simulink model "MI6FS_HE_6PhS"  (R2023a)
settings: Solver=FixedStepAuto  StartTime=0  StopTime=L  FixedStep=Ts  RelTol=1e-3
values from neighbouring files (symbols this model uses):
  A = exp(j*pi/3)    [Parameters.m]
  deg = 0    [Parameters.m]
  FV = 9.8    [Parameters.m]
  J = 0.0243    [Parameters.m]
  Lrr = [((1/3*Lm)+Llr) 1/6*Lm -1/6*Lm -1/3*Lm -1/6*Lm 1/6*Lm;        1/6*Lm ((1/3*Lm)+Llr) 1/6*Lm -1/6*Lm -1/3*Lm -1/6*Lm;        -1/6*Lm 1/6*Lm ((1/3*Lm)+Llr) 1/6*Lm -1/6*Lm -1/3*Lm;        -1/3*Lm -1/6*Lm 1/6*Lm ((1/3*Lm)+Llr) 1/6*Lm -1/6*Lm;        -1/6*Lm -1/3*Lm -1/6*Lm 1/6*Lm ((1/3*Lm)+Llr) 1/6*Lm;        1/6*Lm -1/6*Lm -1/3*Lm -1/6*Lm 1/6*Lm ((1/3*Lm)+Llr)]    [Parameters.m]
  Lrs = transpose(Lsr)    [Parameters.m]
  Lsr = [0 (pi/3) 2*(pi/3) 3*(pi/3) 4*(pi/3) 5*(pi/3);        -(pi/3) 0 (pi/3) 2*(pi/3) 3*(pi/3) 4*(pi/3);        -2*(pi/3) -(pi/3) 0 (pi/3) 2*(pi/3) 3*(pi/3);        -3*(pi/3) -2*(pi/3) -(pi/3) 0 (pi/3) 2*(pi/3);        -4*(pi/3) -3*(pi/3) -2*(pi/3) -(pi/3) 0 (pi/3);        -5*(pi/3) -4*(pi/3) -3*(pi/3) -2*(pi/3) -(pi/3) 0]    [Parameters.m]
  Lss = [((1/3*Lm)+Lls) 1/6*Lm -1/6*Lm -1/3*Lm -1/6*Lm 1/6*Lm;        1/6*Lm ((1/3*Lm)+Lls) 1/6*Lm -1/6*Lm -1/3*Lm -1/6*Lm;        -1/6*Lm 1/6*Lm ((1/3*Lm)+Lls) 1/6*Lm -1/6*Lm -1/3*Lm;        -1/3*Lm -1/6*Lm 1/6*Lm ((1/3*Lm)+Lls) 1/6*Lm -1/6*Lm;        -1/6*Lm -1/3*Lm -1/6*Lm 1/6*Lm ((1/3*Lm)+Lls) 1/6*Lm;        1/6*Lm -1/6*Lm -1/3*Lm -1/6*Lm 1/6*Lm ((1/3*Lm)+Lls)]    [Parameters.m]
  Lto = 0    [Parameters.m]
  Msr = (1/3)*Lm    (= 0.0620333333333)    [Parameters.m]
  p = 2    [Parameters.m]
  Rcore = 811    [Parameters.m]
  Rrr = Rr*eye(6,6)    [Parameters.m]
  Rss = Rs*eye(6,6)    [Parameters.m]
  Tav = 0.23    [Parameters.m]
  Ts = 1/Fs    (= 1e-05)    [Parameters.m]
  Us = sqrt(2)*180    [Parameters.m]
undefined symbols (not defined in the file or in its folder): DiscIntNeverNeededParam, j
libraries: spsFourierLib x84, spsVoltageMeasurementLib x13, spsACVoltageSourceLib x6, spsControlledCurrentSourceLib x6, spsCurrentMeasurementLib x6, spsSeriesRLCBranchLib x6, spsSequenceAnalyzerLib x6, sharedutil x5, eeRmsMeasurement x2, eeGeneralControl x1, spsSequenceAnalyzerPhasorLib x1, spsabctoAlphaBetaZeroLib x1
(part 2 of 3)

== system MI6FS_HE_6PhS/Phase System/Subsystem12 ==
  abc : Inport
  -wt : Subsystem
  Demux : Demux  Outputs=3
  Demux1 : Demux  Outputs=3
  Demux2 : Demux  Outputs=3
  Display : Display
  Display1 : Display
  Display2 : Display
  Divide : Product  Inputs=*/
  Exp : Math
  Gain : Gain  Gain=j
  Gain1 : Gain  Gain=pi/180
  Magnitude-Angle to Complex1 : MagnitudeAngleToComplex
  Minus : Sum  Inputs=+-
  Product : Product
  Scope : Scope
  Sequence Analyzer1 : spsSequenceAnalyzerLib/Sequence Analyzer  Freq=50  n=1  seq=Positive Negative Zero  InInit=[0, 0]  Ts=Ts
  P : Outport
  N : Outport  Port=2
  0 : Outport  Port=3
  |u| : Outport  Port=4
  <u : Outport  Port=5
  wires:
  Product/1 -> Scope/1
  Gain/1 -> Exp/1
  -wt/1(-wt) -> Gain/1
  Exp/1 -> Product/1
  Demux1/1 -> Minus/2
  Demux1/2 -> Minus/1
  Demux2/2 -> Divide/1
  Demux2/1 -> Divide/2
  Minus/1 -> Display2/1
  Divide/1 -> Display1/1
  Demux/3 -> 0/1
  Demux/2 -> N/1, Product/2
  Gain1/1 -> Demux1/1, Magnitude-Angle to Complex1/2
  Demux/1 -> P/1
  abc/1 -> Sequence Analyzer1/1
  Sequence Analyzer1/1 -> |u|/1, Magnitude-Angle to Complex1/1, Demux2/1
  Sequence Analyzer1/2 -> <u/1, Gain1/1
  Magnitude-Angle to Complex1/1 -> Display/1, Demux/1

== system MI6FS_HE_6PhS/Phase System/Subsystem13 ==
  abc : Inport
  -wt : Subsystem
  Demux : Demux  Outputs=3
  Demux1 : Demux  Outputs=3
  Demux2 : Demux  Outputs=3
  Display : Display
  Display1 : Display
  Display2 : Display
  Divide : Product  Inputs=*/
  Exp : Math
  Gain : Gain  Gain=j
  Gain1 : Gain  Gain=pi/180
  Magnitude-Angle to Complex1 : MagnitudeAngleToComplex
  Minus : Sum  Inputs=+-
  Product : Product
  Scope : Scope
  Sequence Analyzer1 : spsSequenceAnalyzerLib/Sequence Analyzer  Freq=50  n=1  seq=Positive Negative Zero  InInit=[0, 0]  Ts=Ts
  P : Outport
  N : Outport  Port=2
  0 : Outport  Port=3
  |u| : Outport  Port=4
  <u : Outport  Port=5
  wires:
  Magnitude-Angle to Complex1/1 -> Demux/1, Display/1
  Sequence Analyzer1/2 -> Gain1/1, <u/1
  Sequence Analyzer1/1 -> Demux2/1, Magnitude-Angle to Complex1/1, |u|/1
  abc/1 -> Sequence Analyzer1/1
  Demux/1 -> P/1
  Gain1/1 -> Magnitude-Angle to Complex1/2, Demux1/1
  Demux/2 -> Product/2, N/1
  Demux/3 -> 0/1
  Divide/1 -> Display1/1
  Minus/1 -> Display2/1
  Demux2/1 -> Divide/2
  Demux2/2 -> Divide/1
  Demux1/2 -> Minus/1
  Demux1/1 -> Minus/2
  Exp/1 -> Product/1
  -wt/1(-wt) -> Gain/1
  Gain/1 -> Exp/1
  Product/1 -> Scope/1

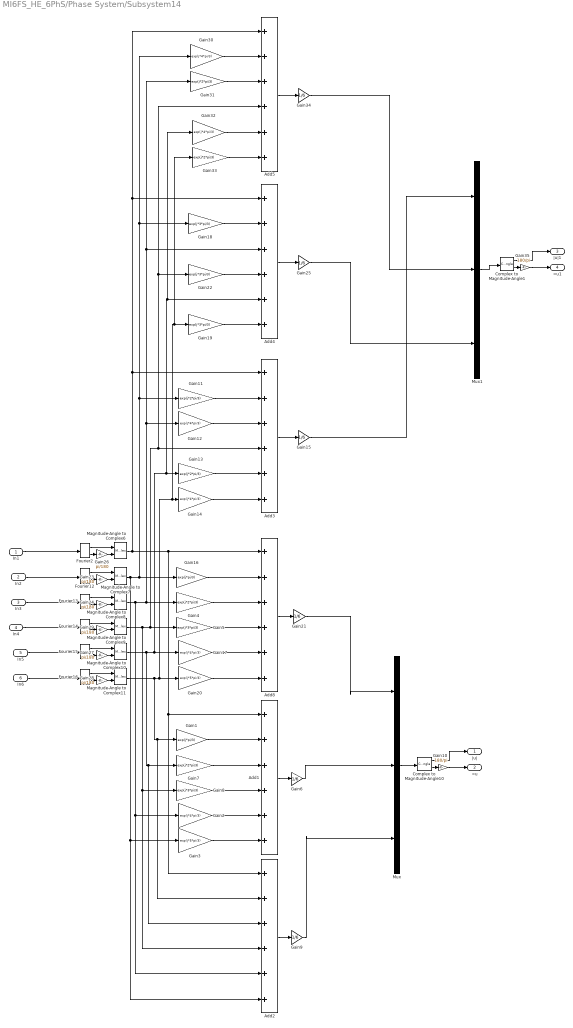
== system MI6FS_HE_6PhS/Phase System/Subsystem14 ==
  In1 : Inport
  In2 : Inport  Port=2
  In3 : Inport  Port=3
  In4 : Inport  Port=4
  In5 : Inport  Port=5
  In6 : Inport  Port=6
  Add{1..5,8} (6 alike) : Sum  Inputs=++++++
  Complex to Magnitude-Angle1 : ComplexToMagnitudeAngle
  Complex to Magnitude-Angle10 : ComplexToMagnitudeAngle
  Fourier{2,12..16} (6 alike) : spsFourierLib/Fourier  Freq=50  n=1  InInit=[0, 0]  Ts=Ts
  Gain1 : Gain  Gain=exp(j*pi/3)
  Gain10 : Gain  Gain=180/pi
  Gain{4,7,11,13,31,33} (6 alike) : Gain  Gain=exp(j*2*pi/3)
  Gain{2,12,14,17,30,32} (6 alike) : Gain  Gain=exp(j*4*pi/3)
  Gain{6,9,15,21,25,34} (6 alike) : Gain  Gain=1/6
  Gain16 : Gain  Gain=exp(j*pi/3)
  Gain{5,8,18..19,22} (5 alike) : Gain  Gain=exp(j*3*pi/3)
  Gain20 : Gain  Gain=exp(j*5*pi/3)
  Gain{23..24,26..29} (6 alike) : Gain  Gain=pi/180
  Gain3 : Gain  Gain=exp(j*5*pi/3)
  Gain35 : Gain  Gain=180/pi
  Magnitude-Angle to Complex{6..11} (6 alike) : MagnitudeAngleToComplex
  Mux : Mux  Inputs=3
  Mux1 : Mux  Inputs=3
  |u| : Outport
  <u : Outport  Port=2
  |u|1 : Outport  Port=3
  <u1 : Outport  Port=4
  wires:
  Gain16/1 -> Add8/2
  Fourier14/2 -> Gain29/1
  Fourier12/2 -> Gain23/1
  Gain27/1 -> Magnitude-Angle to Complex10/2
  Fourier2/2 -> Gain26/1
  Fourier14/1 -> Magnitude-Angle to Complex9/1
  In6/1 -> Fourier16/1
  Magnitude-Angle to Complex7/1 -> Add2/6, Gain3/1, Gain30/1, Gain18/1, Gain11/1, Gain16/1
  Gain28/1 -> Magnitude-Angle to Complex11/2
  In4/1 -> Fourier14/1
  Fourier16/1 -> Magnitude-Angle to Complex11/1
  Fourier2/1 -> Magnitude-Angle to Complex6/1
  Gain4/1 -> Add8/3
  Gain5/1 -> Add8/4
  Magnitude-Angle to Complex10/1 -> Add2/3, Gain7/1, Gain13/1, Gain32/1, Add4/5, Gain17/1
  Magnitude-Angle to Complex9/1 -> Add2/4, Gain8/1, Add5/4, Gain22/1, Add3/4, Gain5/1
  Fourier13/2 -> Gain24/1
  Gain29/1 -> Magnitude-Angle to Complex9/2
  Gain17/1 -> Add8/5
  Gain20/1 -> Add8/6
  In1/1 -> Fourier2/1
  In3/1 -> Fourier13/1
  Fourier16/2 -> Gain28/1
  Fourier15/2 -> Gain27/1
  Fourier15/1 -> Magnitude-Angle to Complex10/1
  Gain23/1 -> Magnitude-Angle to Complex7/2
  Gain24/1 -> Magnitude-Angle to Complex8/2
  Gain26/1 -> Magnitude-Angle to Complex6/2
  Fourier13/1 -> Magnitude-Angle to Complex8/1
  Fourier12/1 -> Magnitude-Angle to Complex7/1
  Add8/1 -> Gain21/1
  Magnitude-Angle to Complex8/1 -> Add2/5, Gain2/1, Gain31/1, Add4/3, Gain12/1, Gain4/1
  In5/1 -> Fourier15/1
  In2/1 -> Fourier12/1
  Gain21/1 -> Mux/1
  Gain3/1 -> Add1/6
  Gain8/1 -> Add1/4
  Gain7/1 -> Add1/3
  Gain2/1 -> Add1/5
  Add1/1 -> Gain6/1
  Gain1/1 -> Add1/2
  Magnitude-Angle to Complex6/1 -> Add5/1, Add4/1, Add3/1, Add2/1, Add1/1, Add8/1
  Gain6/1 -> Mux/2
  Gain9/1 -> Mux/3
  Add2/1 -> Gain9/1
  Complex to Magnitude-Angle10/2 -> Gain10/1
  Mux/1 -> Complex to Magnitude-Angle10/1
  Gain10/1 -> <u/1
  Complex to Magnitude-Angle10/1 -> |u|/1
  Gain11/1 -> Add3/2
  Gain12/1 -> Add3/3
  Gain13/1 -> Add3/5
  Gain14/1 -> Add3/6
  Add3/1 -> Gain15/1
  Gain18/1 -> Add4/2
  Gain22/1 -> Add4/4
  Gain19/1 -> Add4/6
  Add4/1 -> Gain25/1
  Gain30/1 -> Add5/2
  Gain31/1 -> Add5/3
  Gain32/1 -> Add5/5
  Gain33/1 -> Add5/6
  Magnitude-Angle to Complex11/1 -> Add2/2, Gain1/1, Gain19/1, Gain33/1, Gain14/1, Gain20/1
  Add5/1 -> Gain34/1
  Complex to Magnitude-Angle1/1 -> |u|1/1
  Gain35/1 -> <u1/1
  Complex to Magnitude-Angle1/2 -> Gain35/1
  Mux1/1 -> Complex to Magnitude-Angle1/1
  Gain15/1 -> Mux1/1
  Gain34/1 -> Mux1/2
  Gain25/1 -> Mux1/3

== system MI6FS_HE_6PhS/Phase System/Subsystem15 ==
  In1 : Inport
  In2 : Inport  Port=2
  In3 : Inport  Port=3
  Add{1..6} (6 alike) : Sum  Inputs=3
  Add7 : Sum  Inputs=2
  Complex to Magnitude-Angle : ComplexToMagnitudeAngle
  Complex to Magnitude-Angle1 : ComplexToMagnitudeAngle
  Complex to Magnitude-Angle2 : ComplexToMagnitudeAngle
  Display{,1..5} (6 alike) : Display
  Gain{1,5,8,16} (4 alike) : Gain  Gain=exp(j*4*pi/3)
  Gain10 : Gain  Gain=180/pi
  Gain11 : Gain  Gain=180/pi
  Gain12 : Gain  Gain=180/pi
  Gain13 : Gain  Gain=2/3
  Gain{2,4,6,17} (4 alike) : Gain  Gain=exp(j*2*pi/3)
  Gain19 : Gain  Gain=-1/2
  Gain22 : Gain  Gain=2/3
  Gain3 : Gain  Gain=-sqrt(3)/2
  Gain7 : Gain  Gain=-1/2
  Gain9 : Gain  Gain=sqrt(3)/2
  Out1 : Outport
  Out2 : Outport  Port=2
  wires:
  Add1/1 -> Complex to Magnitude-Angle/1, Add6/1
  Gain16/1 -> Add5/2
  In1/1 -> Gain17/1, Gain8/1, Gain2/1, Gain5/1, Add1/1
  Add5/1 -> Complex to Magnitude-Angle2/1, Gain19/1
  In2/1 -> Gain16/1, Gain6/1, Gain1/1, Gain4/1, Add1/2
  Gain17/1 -> Add5/1
  In3/1 -> Add5/3, Add2/3, Add3/3, Add4/3, Add1/3
  Gain4/1 -> Add4/2
  Add4/1 -> Complex to Magnitude-Angle1/1, Gain7/1
  Gain19/1 -> Add6/3
  Gain7/1 -> Add6/2
  Gain5/1 -> Add4/1
  Gain6/1 -> Add2/2
  Gain8/1 -> Add2/1
  Gain1/1 -> Add3/2
  Add3/1 -> Gain3/1
  Gain2/1 -> Add3/1
  Add2/1 -> Gain9/1
  Gain9/1 -> Add7/1
  Gain3/1 -> Add7/2
  Complex to Magnitude-Angle/1 -> Display/1
  Gain10/1 -> Display1/1
  Complex to Magnitude-Angle/2 -> Gain10/1
  Gain11/1 -> Display3/1
  Complex to Magnitude-Angle1/2 -> Gain11/1
  Complex to Magnitude-Angle1/1 -> Display2/1
  Gain12/1 -> Display5/1
  Complex to Magnitude-Angle2/2 -> Gain12/1
  Complex to Magnitude-Angle2/1 -> Display4/1
  Add6/1 -> Gain22/1
  Gain22/1 -> Out1/1
  Gain13/1 -> Out2/1
  Add7/1 -> Gain13/1

== system MI6FS_HE_6PhS/Phase System/Subsystem16 ==
  In1 : Inport
  In2 : Inport  Port=2
  In3 : Inport  Port=3
  In4 : Inport  Port=4
  In5 : Inport  Port=5
  In6 : Inport  Port=6
  Add1 : Sum  Inputs=6
  Display{,2..3,100..111} (15 alike) : Display
  Divide : Product  Inputs=*/
  Fourier{32..37} (6 alike) : spsFourierLib/Fourier  Freq=50  n=1  InInit=[0, 0]  Ts=Ts
  Gain15 : Gain  Gain=1/6
  Max of Elements : MinMax  Function=max
  Minus{,1..5} (6 alike) : Sum  Inputs=+-
  Mux : Mux  Inputs=6
  Out1 : Outport
  Out2 : Outport  Port=2
  wires:
  Fourier32/1 -> Minus1/1, Add1/2, Display102/1
  Fourier32/2 -> Display103/1
  Add1/1 -> Gain15/1
  Fourier33/2 -> Display105/1
  Fourier33/1 -> Minus2/1, Add1/3, Display104/1
  Fourier34/1 -> Display106/1, Minus3/1, Add1/4
  Fourier36/1 -> Display110/1, Minus5/1, Add1/6
  Fourier37/1 -> Display100/1, Minus/1, Add1/1
  Fourier35/1 -> Display108/1, Minus4/1, Add1/5
  In4/1 -> Fourier34/1
  Fourier35/2 -> Display109/1
  Fourier37/2 -> Display101/1
  Fourier36/2 -> Display111/1
  Fourier34/2 -> Display107/1
  Gain15/1 -> Divide/2, Out1/1, [avg]
  In6/1 -> Fourier36/1
  In3/1 -> Fourier33/1
  In5/1 -> Fourier35/1
  In1/1 -> Fourier37/1
  In2/1 -> Fourier32/1
  [avg] -> Minus1/2, Minus/2, Minus2/2, Minus5/2, Minus4/2, Minus3/2
  Mux/1 -> Max of Elements/1, Display2/1
  Minus5/1 -> Mux/6
  Minus4/1 -> Mux/5
  Minus3/1 -> Mux/4
  Minus2/1 -> Mux/3
  Minus1/1 -> Mux/2
  Minus/1 -> Mux/1
  Max of Elements/1 -> Display3/1, Divide/1
  Divide/1 -> Out2/1, Display/1

== system MI6FS_HE_6PhS/Phase System/Subsystem17 ==
  In6 : Inport
  In1 : Inport  Port=2
  In2 : Inport  Port=3
  In3 : Inport  Port=4
  In4 : Inport  Port=5
  In5 : Inport  Port=6
  Add : Sum  Inputs=6
  Add1 : Sum  Inputs=6
  Gain : Gain  Gain=1/3
  Gain1 : Gain  Gain=cos(3*pi/3)
  Gain2 : Gain  Gain=cos(4*pi/3)
  Gain23 : Gain  Gain=cos(pi/3)
  Gain24 : Gain  Gain=cos(2*pi/3)
  Gain3 : Gain  Gain=cos(5*pi/3)
  Gain4 : Gain  Gain=1/3
  Gain5 : Gain  Gain=sin(3*pi/3)
  Gain6 : Gain  Gain=sin(4*pi/3)
  Gain7 : Gain  Gain=sin(pi/3)
  Gain8 : Gain  Gain=sin(2*pi/3)
  Gain9 : Gain  Gain=sin(5*pi/3)
  Out1 : Outport
  Out2 : Outport  Port=2
  wires:
  Gain23/1 -> Add/2
  Gain24/1 -> Add/3
  Add/1 -> Gain/1
  Gain1/1 -> Add/4
  Gain2/1 -> Add/5
  Gain3/1 -> Add/6
  In6/1 -> Add/1
  Gain/1 -> Out1/1
  Gain5/1 -> Add1/4
  In2/1 -> Gain8/1, Gain24/1
  In3/1 -> Gain5/1, Gain1/1
  In5/1 -> Gain9/1, Gain3/1
  In4/1 -> Gain6/1, Gain2/1
  Gain7/1 -> Add1/2
  In1/1 -> Gain7/1, Gain23/1
  Add1/1 -> Gain4/1
  Gain4/1 -> Out2/1
  Gain9/1 -> Add1/6
  Gain8/1 -> Add1/3
  Gain6/1 -> Add1/5

== system MI6FS_HE_6PhS/Phase System/Subsystem18 ==
  In6 : Inport
  In1 : Inport  Port=2
  In2 : Inport  Port=3
  In3 : Inport  Port=4
  In4 : Inport  Port=5
  In5 : Inport  Port=6
  Add : Sum  Inputs=6
  Add1 : Sum  Inputs=6
  Gain : Gain  Gain=1/3
  Gain1 : Gain  Gain=cos(3*pi/3)
  Gain2 : Gain  Gain=cos(4*pi/3)
  Gain23 : Gain  Gain=cos(pi/3)
  Gain24 : Gain  Gain=cos(2*pi/3)
  Gain3 : Gain  Gain=cos(5*pi/3)
  Gain4 : Gain  Gain=1/3
  Gain5 : Gain  Gain=sin(3*pi/3)
  Gain6 : Gain  Gain=sin(4*pi/3)
  Gain7 : Gain  Gain=sin(pi/3)
  Gain8 : Gain  Gain=sin(2*pi/3)
  Gain9 : Gain  Gain=sin(5*pi/3)
  Out1 : Outport
  Out2 : Outport  Port=2
  wires:
  Gain6/1 -> Add1/5
  Gain8/1 -> Add1/3
  Gain9/1 -> Add1/6
  Gain4/1 -> Out2/1
  Add1/1 -> Gain4/1
  In1/1 -> Gain23/1, Gain7/1
  Gain7/1 -> Add1/2
  In4/1 -> Gain2/1, Gain6/1
  In5/1 -> Gain3/1, Gain9/1
  In3/1 -> Gain1/1, Gain5/1
  In2/1 -> Gain24/1, Gain8/1
  Gain5/1 -> Add1/4
  Gain/1 -> Out1/1
  In6/1 -> Add/1
  Gain3/1 -> Add/6
  Gain2/1 -> Add/5
  Gain1/1 -> Add/4
  Add/1 -> Gain/1
  Gain24/1 -> Add/3
  Gain23/1 -> Add/2

== system MI6FS_HE_6PhS/Phase System/Subsystem19 ==
  In1 : Inport
  In2 : Inport  Port=2
  In3 : Inport  Port=3
  In4 : Inport  Port=4
  In5 : Inport  Port=5
  In6 : Inport  Port=6
  Complex to Magnitude-Angle{2..7} (6 alike) : ComplexToMagnitudeAngle
  Constant : Constant  Value=[1 1 1 1 1 1; 1 A A^2 A^3 A^4 A^5; 1 A^2 A^4 1 A^2 A^4; 1 A^3 1 A^3 1 A^3; 1 A^4 A^2 1 A^4 A^2; 1 A^5 A^4 A^3 A^2 A^1]
  Demux : Demux  Outputs=6
  Display{2..11} (10 alike) : Display
  Fourier{2,12..16} (6 alike) : spsFourierLib/Fourier  Freq=50  n=1  InInit=[0, 0]  Ts=Ts
  Gain : Gain  Gain=1/6
  Gain{2..6,43} (6 alike) : Gain  Gain=180/pi
  Gain{23..24,26..29} (6 alike) : Gain  Gain=pi/180
  Magnitude-Angle to Complex{6..11} (6 alike) : MagnitudeAngleToComplex
  Matrix Multiply : Product  Multiplication=Matrix(*)
  Mux : Mux  Inputs=6
  Subsystem : Subsystem
  |u| : Outport
  <u : Outport  Port=2
  wires:
  Fourier14/2 -> Gain29/1
  Fourier12/2 -> Gain23/1
  Gain27/1 -> Magnitude-Angle to Complex10/2
  Fourier2/2 -> Gain26/1
  Fourier14/1 -> Magnitude-Angle to Complex9/1
  In6/1 -> Fourier16/1
  Gain28/1 -> Magnitude-Angle to Complex11/2
  In4/1 -> Fourier14/1
  Fourier16/1 -> Magnitude-Angle to Complex11/1
  Fourier2/1 -> Magnitude-Angle to Complex6/1
  Fourier13/2 -> Gain24/1
  Gain29/1 -> Magnitude-Angle to Complex9/2
  In1/1 -> Fourier2/1
  In3/1 -> Fourier13/1
  Fourier16/2 -> Gain28/1
  Fourier15/2 -> Gain27/1
  Fourier15/1 -> Magnitude-Angle to Complex10/1
  Gain23/1 -> Magnitude-Angle to Complex7/2
  Gain24/1 -> Magnitude-Angle to Complex8/2
  Gain26/1 -> Magnitude-Angle to Complex6/2
  Fourier13/1 -> Magnitude-Angle to Complex8/1
  Fourier12/1 -> Magnitude-Angle to Complex7/1
  In5/1 -> Fourier15/1
  In2/1 -> Fourier12/1
  Gain2/1 -> Display3/1
  Complex to Magnitude-Angle4/1 -> Display4/1
  Complex to Magnitude-Angle4/2 -> Gain3/1
  Gain3/1 -> Display5/1
  Demux/1 -> Subsystem/1(U0)
  Gain4/1 -> Display7/1
  Demux/4 -> Subsystem/4(U20)
  Subsystem/6(Unab) -> Complex to Magnitude-Angle7/1
  Complex to Magnitude-Angle3/1 -> Display2/1
  Subsystem/5(U2nab) -> Complex to Magnitude-Angle6/1
  Demux/2 -> Subsystem/2(Up)
  Demux/5 -> Subsystem/5(U2n)
  Subsystem/3(U2pab) -> Complex to Magnitude-Angle4/1
  Complex to Magnitude-Angle7/2 -> Gain6/1
  Complex to Magnitude-Angle7/1 -> Display10/1
  Subsystem/4(U20ab) -> Complex to Magnitude-Angle5/1
  Matrix Multiply/1 -> Gain/1
  Gain6/1 -> Display11/1
  Mux/1 -> Matrix Multiply/2
  Constant/1 -> Matrix Multiply/1
  Complex to Magnitude-Angle6/2 -> Gain5/1
  Complex to Magnitude-Angle6/1 -> Display8/1
  Gain5/1 -> Display9/1
  Demux/6 -> Subsystem/6(Un)
  Complex to Magnitude-Angle5/2 -> Gain4/1
  Complex to Magnitude-Angle2/2 -> Gain43/1
  Demux/3 -> Subsystem/3(U2p)
  Complex to Magnitude-Angle2/1 -> |u|/1
  Gain43/1 -> <u/1
  Subsystem/2(Upab) -> Complex to Magnitude-Angle3/1
  Complex to Magnitude-Angle5/1 -> Display6/1
  Complex to Magnitude-Angle3/2 -> Gain2/1
  Gain/1 -> Demux/1, Complex to Magnitude-Angle2/1
  Magnitude-Angle to Complex6/1 -> Mux/1
  Magnitude-Angle to Complex7/1 -> Mux/2
  Magnitude-Angle to Complex8/1 -> Mux/3
  Magnitude-Angle to Complex9/1 -> Mux/4
  Magnitude-Angle to Complex10/1 -> Mux/5
  Magnitude-Angle to Complex11/1 -> Mux/6

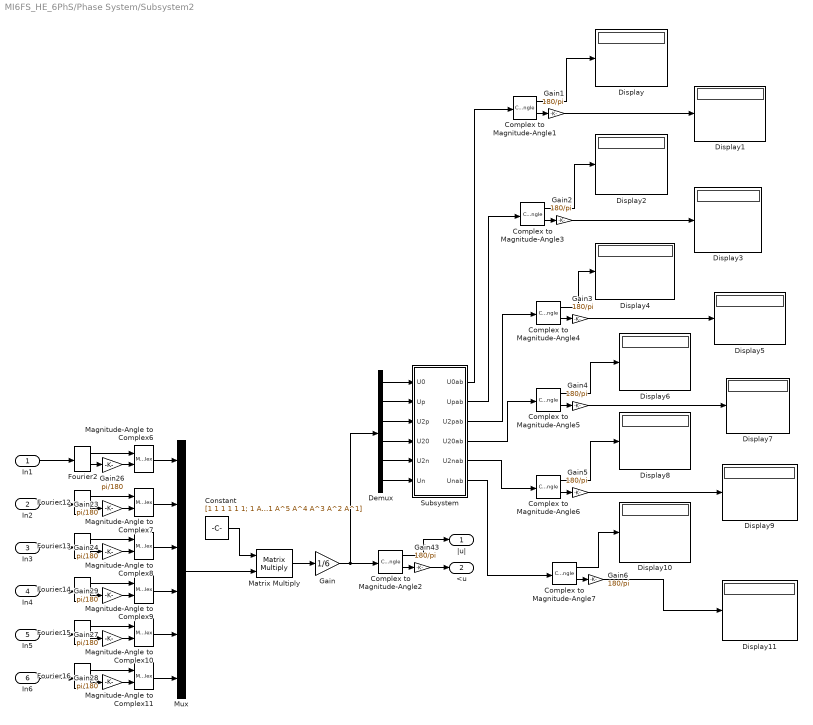
== system MI6FS_HE_6PhS/Phase System/Subsystem2 ==
  In1 : Inport
  In2 : Inport  Port=2
  In3 : Inport  Port=3
  In4 : Inport  Port=4
  In5 : Inport  Port=5
  In6 : Inport  Port=6
  Complex to Magnitude-Angle{1..7} (7 alike) : ComplexToMagnitudeAngle
  Constant : Constant  Value=[1 1 1 1 1 1; 1 A A^2 A^3 A^4 A^5; 1 A^2 A^4 1 A^2 A^4; 1 A^3 1 A^3 1 A^3; 1 A^4 A^2 1 A^4 A^2; 1 A^5 A^4 A^3 A^2 A^1]
  Demux : Demux  Outputs=6
  Display{,1..11} (12 alike) : Display
  Fourier{2,12..16} (6 alike) : spsFourierLib/Fourier  Freq=50  n=1  InInit=[0, 0]  Ts=Ts
  Gain : Gain  Gain=1/6
  Gain{1..6,43} (7 alike) : Gain  Gain=180/pi
  Gain{23..24,26..29} (6 alike) : Gain  Gain=pi/180
  Magnitude-Angle to Complex{6..11} (6 alike) : MagnitudeAngleToComplex
  Matrix Multiply : Product  Multiplication=Matrix(*)
  Mux : Mux  Inputs=6
  Subsystem : Subsystem
  |u| : Outport
  <u : Outport  Port=2
  wires:
  Fourier14/2 -> Gain29/1
  Fourier12/2 -> Gain23/1
  Gain27/1 -> Magnitude-Angle to Complex10/2
  Fourier2/2 -> Gain26/1
  Fourier14/1 -> Magnitude-Angle to Complex9/1
  In6/1 -> Fourier16/1
  Gain28/1 -> Magnitude-Angle to Complex11/2
  In4/1 -> Fourier14/1
  Fourier16/1 -> Magnitude-Angle to Complex11/1
  Fourier2/1 -> Magnitude-Angle to Complex6/1
  Fourier13/2 -> Gain24/1
  Gain29/1 -> Magnitude-Angle to Complex9/2
  In1/1 -> Fourier2/1
  In3/1 -> Fourier13/1
  Fourier16/2 -> Gain28/1
  Fourier15/2 -> Gain27/1
  Fourier15/1 -> Magnitude-Angle to Complex10/1
  Gain23/1 -> Magnitude-Angle to Complex7/2
  Gain24/1 -> Magnitude-Angle to Complex8/2
  Gain26/1 -> Magnitude-Angle to Complex6/2
  Fourier13/1 -> Magnitude-Angle to Complex8/1
  Fourier12/1 -> Magnitude-Angle to Complex7/1
  In5/1 -> Fourier15/1
  In2/1 -> Fourier12/1
  Complex to Magnitude-Angle1/1 -> Display/1
  Gain2/1 -> Display3/1
  Complex to Magnitude-Angle4/1 -> Display4/1
  Complex to Magnitude-Angle4/2 -> Gain3/1
  Gain3/1 -> Display5/1
  Demux/1 -> Subsystem/1(U0)
  Gain4/1 -> Display7/1
  Demux/4 -> Subsystem/4(U20)
  Subsystem/6(Unab) -> Complex to Magnitude-Angle7/1
  Complex to Magnitude-Angle3/1 -> Display2/1
  Subsystem/5(U2nab) -> Complex to Magnitude-Angle6/1
  Demux/2 -> Subsystem/2(Up)
  Demux/5 -> Subsystem/5(U2n)
  Subsystem/3(U2pab) -> Complex to Magnitude-Angle4/1
  Complex to Magnitude-Angle7/2 -> Gain6/1
  Complex to Magnitude-Angle7/1 -> Display10/1
  Subsystem/4(U20ab) -> Complex to Magnitude-Angle5/1
  Matrix Multiply/1 -> Gain/1
  Gain6/1 -> Display11/1
  Mux/1 -> Matrix Multiply/2
  Constant/1 -> Matrix Multiply/1
  Complex to Magnitude-Angle6/2 -> Gain5/1
  Complex to Magnitude-Angle6/1 -> Display8/1
  Gain5/1 -> Display9/1
  Gain1/1 -> Display1/1
  Demux/6 -> Subsystem/6(Un)
  Subsystem/1(U0ab) -> Complex to Magnitude-Angle1/1
  Complex to Magnitude-Angle5/2 -> Gain4/1
  Complex to Magnitude-Angle2/2 -> Gain43/1
  Demux/3 -> Subsystem/3(U2p)
  Complex to Magnitude-Angle2/1 -> |u|/1
  Gain43/1 -> <u/1
  Subsystem/2(Upab) -> Complex to Magnitude-Angle3/1
  Complex to Magnitude-Angle5/1 -> Display6/1
  Complex to Magnitude-Angle3/2 -> Gain2/1
  Complex to Magnitude-Angle1/2 -> Gain1/1
  Gain/1 -> Demux/1, Complex to Magnitude-Angle2/1
  Magnitude-Angle to Complex6/1 -> Mux/1
  Magnitude-Angle to Complex7/1 -> Mux/2
  Magnitude-Angle to Complex8/1 -> Mux/3
  Magnitude-Angle to Complex9/1 -> Mux/4
  Magnitude-Angle to Complex10/1 -> Mux/5
  Magnitude-Angle to Complex11/1 -> Mux/6

== system MI6FS_HE_6PhS/Phase System/Subsystem20 ==
  In1 : Inport
  In2 : Inport  Port=2
  In3 : Inport  Port=3
  In4 : Inport  Port=4
  In5 : Inport  Port=5
  In6 : Inport  Port=6
  Complex to Magnitude-Angle{2..7} (6 alike) : ComplexToMagnitudeAngle
  Constant : Constant  Value=[1 1 1 1 1 1; 1 A A^2 A^3 A^4 A^5; 1 A^2 A^4 1 A^2 A^4; 1 A^3 1 A^3 1 A^3; 1 A^4 A^2 1 A^4 A^2; 1 A^5 A^4 A^3 A^2 A^1]
  Demux : Demux  Outputs=6
  Display{2..11} (10 alike) : Display
  Fourier{2,12..16} (6 alike) : spsFourierLib/Fourier  Freq=50  n=1  InInit=[0, 0]  Ts=Ts
  Gain : Gain  Gain=1/6
  Gain{2..6,43} (6 alike) : Gain  Gain=180/pi
  Gain{23..24,26..29} (6 alike) : Gain  Gain=pi/180
  Magnitude-Angle to Complex{6..11} (6 alike) : MagnitudeAngleToComplex
  Matrix Multiply : Product  Multiplication=Matrix(*)
  Mux : Mux  Inputs=6
  Subsystem : Subsystem
  |u| : Outport
  <u : Outport  Port=2
  wires:
  Magnitude-Angle to Complex11/1 -> Mux/6
  Magnitude-Angle to Complex10/1 -> Mux/5
  Magnitude-Angle to Complex9/1 -> Mux/4
  Magnitude-Angle to Complex8/1 -> Mux/3
  Magnitude-Angle to Complex7/1 -> Mux/2
  Magnitude-Angle to Complex6/1 -> Mux/1
  Gain/1 -> Complex to Magnitude-Angle2/1, Demux/1
  Complex to Magnitude-Angle3/2 -> Gain2/1
  Complex to Magnitude-Angle5/1 -> Display6/1
  Subsystem/2(Upab) -> Complex to Magnitude-Angle3/1
  Gain43/1 -> <u/1
  Complex to Magnitude-Angle2/1 -> |u|/1
  Demux/3 -> Subsystem/3(U2p)
  Complex to Magnitude-Angle2/2 -> Gain43/1
  Complex to Magnitude-Angle5/2 -> Gain4/1
  Demux/6 -> Subsystem/6(Un)
  Gain5/1 -> Display9/1
  Complex to Magnitude-Angle6/1 -> Display8/1
  Complex to Magnitude-Angle6/2 -> Gain5/1
  Constant/1 -> Matrix Multiply/1
  Mux/1 -> Matrix Multiply/2
  Gain6/1 -> Display11/1
  Matrix Multiply/1 -> Gain/1
  Subsystem/4(U20ab) -> Complex to Magnitude-Angle5/1
  Complex to Magnitude-Angle7/1 -> Display10/1
  Complex to Magnitude-Angle7/2 -> Gain6/1
  Subsystem/3(U2pab) -> Complex to Magnitude-Angle4/1
  Demux/5 -> Subsystem/5(U2n)
  Demux/2 -> Subsystem/2(Up)
  Subsystem/5(U2nab) -> Complex to Magnitude-Angle6/1
  Complex to Magnitude-Angle3/1 -> Display2/1
  Subsystem/6(Unab) -> Complex to Magnitude-Angle7/1
  Demux/4 -> Subsystem/4(U20)
  Gain4/1 -> Display7/1
  Demux/1 -> Subsystem/1(U0)
  Gain3/1 -> Display5/1
  Complex to Magnitude-Angle4/2 -> Gain3/1
  Complex to Magnitude-Angle4/1 -> Display4/1
  Gain2/1 -> Display3/1
  In2/1 -> Fourier12/1
  In5/1 -> Fourier15/1
  Fourier12/1 -> Magnitude-Angle to Complex7/1
  Fourier13/1 -> Magnitude-Angle to Complex8/1
  Gain26/1 -> Magnitude-Angle to Complex6/2
  Gain24/1 -> Magnitude-Angle to Complex8/2
  Gain23/1 -> Magnitude-Angle to Complex7/2
  Fourier15/1 -> Magnitude-Angle to Complex10/1
  Fourier15/2 -> Gain27/1
  Fourier16/2 -> Gain28/1
  In3/1 -> Fourier13/1
  In1/1 -> Fourier2/1
  Gain29/1 -> Magnitude-Angle to Complex9/2
  Fourier13/2 -> Gain24/1
  Fourier2/1 -> Magnitude-Angle to Complex6/1
  Fourier16/1 -> Magnitude-Angle to Complex11/1
  In4/1 -> Fourier14/1
  Gain28/1 -> Magnitude-Angle to Complex11/2
  In6/1 -> Fourier16/1
  Fourier14/1 -> Magnitude-Angle to Complex9/1
  Fourier2/2 -> Gain26/1
  Gain27/1 -> Magnitude-Angle to Complex10/2
  Fourier12/2 -> Gain23/1
  Fourier14/2 -> Gain29/1

== system MI6FS_HE_6PhS/Phase System/Subsystem21 ==
  In1 : Inport
  In2 : Inport  Port=2
  In3 : Inport  Port=3
  In4 : Inport  Port=4
  In5 : Inport  Port=5
  In6 : Inport  Port=6
  Complex to Magnitude-Angle{2..7} (6 alike) : ComplexToMagnitudeAngle
  Constant : Constant  Value=[1 1 1 1 1 1; 1 A A^2 A^3 A^4 A^5; 1 A^2 A^4 1 A^2 A^4; 1 A^3 1 A^3 1 A^3; 1 A^4 A^2 1 A^4 A^2; 1 A^5 A^4 A^3 A^2 A^1]
  Demux : Demux  Outputs=6
  Display{2..11} (10 alike) : Display
  Fourier{2,12..16} (6 alike) : spsFourierLib/Fourier  Freq=50  n=1  InInit=[0, 0]  Ts=Ts
  Gain : Gain  Gain=1/6
  Gain{2..6,43} (6 alike) : Gain  Gain=180/pi
  Gain{23..24,26..29} (6 alike) : Gain  Gain=pi/180
  Magnitude-Angle to Complex{6..11} (6 alike) : MagnitudeAngleToComplex
  Matrix Multiply : Product  Multiplication=Matrix(*)
  Mux : Mux  Inputs=6
  Subsystem : Subsystem
  |u| : Outport
  <u : Outport  Port=2
  wires:
  Magnitude-Angle to Complex11/1 -> Mux/6
  Magnitude-Angle to Complex10/1 -> Mux/5
  Magnitude-Angle to Complex9/1 -> Mux/4
  Magnitude-Angle to Complex8/1 -> Mux/3
  Magnitude-Angle to Complex7/1 -> Mux/2
  Magnitude-Angle to Complex6/1 -> Mux/1
  Gain/1 -> Complex to Magnitude-Angle2/1, Demux/1
  Complex to Magnitude-Angle3/2 -> Gain2/1
  Complex to Magnitude-Angle5/1 -> Display6/1
  Subsystem/2(Upab) -> Complex to Magnitude-Angle3/1
  Gain43/1 -> <u/1
  Complex to Magnitude-Angle2/1 -> |u|/1
  Demux/3 -> Subsystem/3(U2p)
  Complex to Magnitude-Angle2/2 -> Gain43/1
  Complex to Magnitude-Angle5/2 -> Gain4/1
  Demux/6 -> Subsystem/6(Un)
  Gain5/1 -> Display9/1
  Complex to Magnitude-Angle6/1 -> Display8/1
  Complex to Magnitude-Angle6/2 -> Gain5/1
  Constant/1 -> Matrix Multiply/1
  Mux/1 -> Matrix Multiply/2
  Gain6/1 -> Display11/1
  Matrix Multiply/1 -> Gain/1
  Subsystem/4(U20ab) -> Complex to Magnitude-Angle5/1
  Complex to Magnitude-Angle7/1 -> Display10/1
  Complex to Magnitude-Angle7/2 -> Gain6/1
  Subsystem/3(U2pab) -> Complex to Magnitude-Angle4/1
  Demux/5 -> Subsystem/5(U2n)
  Demux/2 -> Subsystem/2(Up)
  Subsystem/5(U2nab) -> Complex to Magnitude-Angle6/1
  Complex to Magnitude-Angle3/1 -> Display2/1
  Subsystem/6(Unab) -> Complex to Magnitude-Angle7/1
  Demux/4 -> Subsystem/4(U20)
  Gain4/1 -> Display7/1
  Demux/1 -> Subsystem/1(U0)
  Gain3/1 -> Display5/1
  Complex to Magnitude-Angle4/2 -> Gain3/1
  Complex to Magnitude-Angle4/1 -> Display4/1
  Gain2/1 -> Display3/1
  In2/1 -> Fourier12/1
  In5/1 -> Fourier15/1
  Fourier12/1 -> Magnitude-Angle to Complex7/1
  Fourier13/1 -> Magnitude-Angle to Complex8/1
  Gain26/1 -> Magnitude-Angle to Complex6/2
  Gain24/1 -> Magnitude-Angle to Complex8/2
  Gain23/1 -> Magnitude-Angle to Complex7/2
  Fourier15/1 -> Magnitude-Angle to Complex10/1
  Fourier15/2 -> Gain27/1
  Fourier16/2 -> Gain28/1
  In3/1 -> Fourier13/1
  In1/1 -> Fourier2/1
  Gain29/1 -> Magnitude-Angle to Complex9/2
  Fourier13/2 -> Gain24/1
  Fourier2/1 -> Magnitude-Angle to Complex6/1
  Fourier16/1 -> Magnitude-Angle to Complex11/1
  In4/1 -> Fourier14/1
  Gain28/1 -> Magnitude-Angle to Complex11/2
  In6/1 -> Fourier16/1
  Fourier14/1 -> Magnitude-Angle to Complex9/1
  Fourier2/2 -> Gain26/1
  Gain27/1 -> Magnitude-Angle to Complex10/2
  Fourier12/2 -> Gain23/1
  Fourier14/2 -> Gain29/1

== system MI6FS_HE_6PhS/Phase System/Subsystem3 ==
  abc : Inport
  -wt : Subsystem
  Demux : Demux  Outputs=3
  Demux1 : Demux  Outputs=3
  Demux2 : Demux  Outputs=3
  Display : Display
  Display1 : Display
  Display2 : Display
  Divide : Product  Inputs=*/
  Exp : Math
  Gain : Gain  Gain=j
  Gain1 : Gain  Gain=pi/180
  Magnitude-Angle to Complex1 : MagnitudeAngleToComplex
  Minus : Sum  Inputs=+-
  Product : Product
  Scope : Scope
  Sequence Analyzer1 : spsSequenceAnalyzerLib/Sequence Analyzer  Freq=50  n=1  seq=Positive Negative Zero  InInit=[0, 0]  Ts=Ts
  P : Outport
  N : Outport  Port=2
  0 : Outport  Port=3
  |u| : Outport  Port=4
  <u : Outport  Port=5
  wires:
  Magnitude-Angle to Complex1/1 -> Demux/1, Display/1
  Sequence Analyzer1/2 -> Gain1/1, <u/1
  Sequence Analyzer1/1 -> Demux2/1, Magnitude-Angle to Complex1/1, |u|/1
  abc/1 -> Sequence Analyzer1/1
  Demux/1 -> P/1
  Gain1/1 -> Magnitude-Angle to Complex1/2, Demux1/1
  Demux/2 -> Product/2, N/1
  Demux/3 -> 0/1
  Divide/1 -> Display1/1
  Minus/1 -> Display2/1
  Demux2/1 -> Divide/2
  Demux2/2 -> Divide/1
  Demux1/2 -> Minus/1
  Demux1/1 -> Minus/2
  Exp/1 -> Product/1
  -wt/1(-wt) -> Gain/1
  Gain/1 -> Exp/1
  Product/1 -> Scope/1

== system MI6FS_HE_6PhS/Phase System/Subsystem4 ==
  P : Inport
  N : Inport  Port=2
  Complex to Magnitude-Angle2 : ComplexToMagnitudeAngle
  Divide1 : Product  Inputs=*/
  Gain1 : Gain  Gain=180/pi
  K : Outport
  phase : Outport  Port=2
  wires:
  Gain1/1 -> phase/1
  Complex to Magnitude-Angle2/1 -> K/1
  Divide1/1 -> Complex to Magnitude-Angle2/1
  Complex to Magnitude-Angle2/2 -> Gain1/1
  N/1 -> Divide1/1
  P/1 -> Divide1/2

== system MI6FS_HE_6PhS/Phase System/Subsystem5 ==
  abc : Inport
  -wt : Subsystem
  Demux : Demux  Outputs=3
  Display : Display
  Exp : Math
  Gain : Gain  Gain=j
  Gain1 : Gain  Gain=pi/180
  Magnitude-Angle to Complex1 : MagnitudeAngleToComplex
  Product : Product
  Scope : Scope
  Sequence Analyzer1 : spsSequenceAnalyzerLib/Sequence Analyzer  Freq=50  n=1  seq=Positive Negative Zero  InInit=[0, 0]  Ts=Ts
  P : Outport
  N : Outport  Port=2
  0 : Outport  Port=3
  |u| : Outport  Port=4
  <u : Outport  Port=5
  wires:
  Demux/3 -> 0/1
  Gain1/1 -> Magnitude-Angle to Complex1/2
  abc/1 -> Sequence Analyzer1/1
  Sequence Analyzer1/1 -> |u|/1, Magnitude-Angle to Complex1/1
  Sequence Analyzer1/2 -> <u/1, Gain1/1
  Magnitude-Angle to Complex1/1 -> Demux/1, Display/1
  Demux/1 -> P/1
  -wt/1(-wt) -> Gain/1
  Exp/1 -> Product/1
  Product/1 -> Scope/1
  Gain/1 -> Exp/1
  Demux/2 -> Product/2, N/1

== system MI6FS_HE_6PhS/Phase System/Subsystem6 ==
  abc : Inport
  Demux : Demux  Outputs=3
  Display : Display
  Gain1 : Gain  Gain=pi/180
  Magnitude-Angle to Complex1 : MagnitudeAngleToComplex
  Sequence Analyzer1 : spsSequenceAnalyzerLib/Sequence Analyzer  Freq=50  n=1  seq=Positive Negative Zero  InInit=[0, 0]  Ts=Ts
  P : Outport
  N : Outport  Port=2
  0 : Outport  Port=3
  |u| : Outport  Port=4
  <u : Outport  Port=5
  wires:
  Magnitude-Angle to Complex1/1 -> Display/1, Demux/1
  Sequence Analyzer1/2 -> Gain1/1, <u/1
  Sequence Analyzer1/1 -> Magnitude-Angle to Complex1/1, |u|/1
  abc/1 -> Sequence Analyzer1/1
  Gain1/1 -> Magnitude-Angle to Complex1/2
  Demux/3 -> 0/1
  Demux/1 -> P/1
  Demux/2 -> N/1

== system MI6FS_HE_6PhS/Phase System/Subsystem7 ==
  abc : Inport
  Demux : Demux  Outputs=3
  Display : Display
  Gain1 : Gain  Gain=pi/180
  Magnitude-Angle to Complex1 : MagnitudeAngleToComplex
  Sequence Analyzer1 : spsSequenceAnalyzerLib/Sequence Analyzer  Freq=50  n=1  seq=Positive Negative Zero  InInit=[0, 0]  Ts=Ts
  P : Outport
  N : Outport  Port=2
  0 : Outport  Port=3
  |u| : Outport  Port=4
  <u : Outport  Port=5
  wires:
  Magnitude-Angle to Complex1/1 -> Display/1, Demux/1
  Sequence Analyzer1/2 -> Gain1/1, <u/1
  Sequence Analyzer1/1 -> Magnitude-Angle to Complex1/1, |u|/1
  abc/1 -> Sequence Analyzer1/1
  Gain1/1 -> Magnitude-Angle to Complex1/2
  Demux/3 -> 0/1
  Demux/1 -> P/1
  Demux/2 -> N/1

== system MI6FS_HE_6PhS/Phase System/Subsystem8 ==
  abc : Inport
  Demux : Demux  Outputs=3
  Display : Display
  Gain1 : Gain  Gain=pi/180
  Magnitude-Angle to Complex1 : MagnitudeAngleToComplex
  Sequence Analyzer (Phasor) : spsSequenceAnalyzerPhasorLib/Sequence Analyzer (Phasor)  seq=Positive Negative Zero
  P : Outport
  N : Outport  Port=2
  0 : Outport  Port=3
  |u| : Outport  Port=4
  <u : Outport  Port=5
  wires:
  Demux/2 -> N/1
  Demux/1 -> P/1
  Demux/3 -> 0/1
  Gain1/1 -> Magnitude-Angle to Complex1/2
  abc/1 -> Sequence Analyzer (Phasor)/1
  Sequence Analyzer (Phasor)/1 -> |u|/1, Magnitude-Angle to Complex1/1
  Sequence Analyzer (Phasor)/2 -> <u/1, Gain1/1
  Magnitude-Angle to Complex1/1 -> Demux/1, Display/1

== system MI6FS_HE_6PhS/Phase System/Subsystem9 ==
  P : Inport
  N : Inport  Port=2
  Complex to Magnitude-Angle2 : ComplexToMagnitudeAngle
  Divide1 : Product  Inputs=*/
  Gain1 : Gain  Gain=180/pi
  K : Outport
  phase : Outport  Port=2
  wires:
  Gain1/1 -> phase/1
  Complex to Magnitude-Angle2/1 -> K/1
  Divide1/1 -> Complex to Magnitude-Angle2/1
  Complex to Magnitude-Angle2/2 -> Gain1/1
  N/1 -> Divide1/1
  P/1 -> Divide1/2

== system MI6FS_HE_6PhS/Motor System/MOTOR SYSTEM EQUATIONS /ROTOR SYSTEM ==
  note: d/dt [Ir] = 1/[Lrr] * ( [0] - [Rr].[Ir] - (d/dt[Lrs]).[Is] - [Lrs]. d/dt [Is] )
  I_s : Inport
  d/dt I_s : Inport  Port=2
  Teta_R : Inport  Port=3
  We : Inport  Port=4
  Add1 : Sum
  Constant2 : Constant  Value=0
  Constant3 : Constant  Value=Lrs
  Cos1 : Trigonometry  Operator=cos
  Discrete-Time Integrator : DiscreteIntegrator  IntegratorMethod=Integration: Trapezoidal  SampleTime=Ts  ICPrevOutput=DiscIntNeverNeededParam  ICPrevScaledInput=DiscIntNeverNeededParam
  Gain : Gain  Gain=inv(Lrr)  Multiplication=Matrix(K*u)
  Gain1 : Gain  Gain=-Msr  Multiplication=Matrix(K*u)
  Gain4 : Gain  Gain=Rrr  Multiplication=Matrix(K*u)
  Gain8 : Gain  Gain=Msr  Multiplication=Matrix(K*u)
  Product : Product
  Product4 : Product  Multiplication=Matrix(*)
  Product5 : Product  Multiplication=Matrix(*)
  Sin1 : Trigonometry
  Subtract : Sum  Inputs=+-
  Subtract2 : Sum  Inputs=+-
  Subtract3 : Sum  Inputs=+-
  Unit Delay : UnitDelay  SampleTime=Ts  HasFrameUpgradeWarning=on
  Unit Delay1 : UnitDelay  SampleTime=Ts  HasFrameUpgradeWarning=on
  Unit Delay2 : UnitDelay  SampleTime=Ts  HasFrameUpgradeWarning=on
  Vector Concatenate : Concatenate  NumInputs=6  Mode=Multidimensional array
  I_r : Outport  VectorParamsAs1DForOutWhenUnconnected=off
  d/dt I_r : Outport  Port=2  VectorParamsAs1DForOutWhenUnconnected=off
  wires:
  Cos1/1 -> Gain8/1
  Subtract3/1 -> Subtract/1
  Subtract2/1 -> Subtract3/1  "0-Rr * Ir"
  Gain4/1 -> Subtract2/2
  Add1/1 -> Sin1/1, Cos1/1
  Discrete-Time Integrator/1 -> I_r/1, Unit Delay1/1  "Ir"
  Gain/1 -> Discrete-Time Integrator/1, d/dt I_r/1  "dt/d Ir"
  I_s/1 -> Product4/2  "I_s"
  Vector Concatenate/1 -> Subtract2/1
  Gain8/1 -> Product5/1  "Lrs"
  Subtract/1 -> Gain/1
  Product5/1 -> Unit Delay/1
  Constant3/1 -> Add1/1
  d/dt I_s/1 -> Product5/2
  Unit Delay/1 -> Subtract/2  "Lrs * d/dt Is"
  Product4/1 -> Unit Delay2/1  "d/dt Lrs * Is"
  Gain1/1 -> Product4/1  "d/dt Lrs"
  Constant2/1 -> Vector Concatenate/2, Vector Concatenate/1, Vector Concatenate/3, Vector Concatenate/4, Vector Concatenate/5, Vector Concatenate/6
  Teta_R/1 -> Add1/2
  Product/1 -> Gain1/1
  Sin1/1 -> Product/1
  We/1 -> Product/2
  Unit Delay1/1 -> Gain4/1  "Lrs * d/dt Is"
  Unit Delay2/1 -> Subtract3/2  "Lrs * d/dt Is"

== system MI6FS_HE_6PhS/Motor System/MOTOR SYSTEM EQUATIONS /STATOR SYSTEM ==
  note: d/dt [Is] = 1/[Lss] * ( [Vs] - [Rs].[Is] - (d/dt[Lsr]).[Ir] - [Lsr]. d/dt [Ir] )
  Us-6 : Inport
  I_r : Inport  Port=2
  d/dt I_r : Inport  Port=3
  Teta_R : Inport  Port=4
  We : Inport  Port=5
  Add : Sum
  Constant : Constant  Value=Lsr
  Cos : Trigonometry  Operator=cos
  Discrete-Time Integrator : DiscreteIntegrator  IntegratorMethod=Integration: Trapezoidal  SampleTime=Ts  ICPrevOutput=DiscIntNeverNeededParam  ICPrevScaledInput=DiscIntNeverNeededParam
  Gain : Gain  Gain=Rss  Multiplication=Matrix(K*u)
  Gain3 : Gain  Gain=inv(Lss)  Multiplication=Matrix(K*u)
  Gain4 : Gain  Gain=-Msr  Multiplication=Matrix(K*u)
  Gain7 : Gain  Gain=Msr  Multiplication=Matrix(K*u)
  Product : Product
  Product1 : Product  Multiplication=Matrix(*)
  Product2 : Product  Multiplication=Matrix(*)
  Sin : Trigonometry  OutputSignalType=real
  Subtract : Sum  Inputs=+-
  Subtract1 : Sum  Inputs=+-
  Subtract2 : Sum  Inputs=+-
  Unit Delay : UnitDelay  SampleTime=Ts  HasFrameUpgradeWarning=on
  Unit Delay1 : UnitDelay  SampleTime=Ts  HasFrameUpgradeWarning=on
  Unit Delay2 : UnitDelay  SampleTime=Ts  HasFrameUpgradeWarning=on
  I_s : Outport  VectorParamsAs1DForOutWhenUnconnected=off
  d/dt I_s : Outport  Port=2  VectorParamsAs1DForOutWhenUnconnected=off
  wires:
  I_r/1 -> Product1/2  "Ir"
  Constant/1 -> Add/1
  Add/1 -> Sin/1, Cos/1
  Product2/1 -> Unit Delay/1  "Lsr * d/dt Ir"
  Subtract/1 -> Subtract1/1  "Us - Rs * Is"
  Cos/1 -> Gain7/1
  Gain3/1 -> Discrete-Time Integrator/1, d/dt I_s/1  "d/dt I_s"
  Us-6/1 -> Subtract/1
  Discrete-Time Integrator/1 -> Unit Delay1/1, I_s/1  "Is"
  Gain/1 -> Subtract/2  "Rss * Is"
  Gain7/1 -> Product2/1  "Lsr"
  d/dt I_r/1 -> Product2/2  "d/dt Ir"
  Subtract1/1 -> Subtract2/1
  Subtract2/1 -> Gain3/1
  Unit Delay/1 -> Subtract2/2
  Product1/1 -> Unit Delay2/1  "d/dt Lsr * Ir"
  Gain4/1 -> Product1/1  "d/dt Lsr"
  Teta_R/1 -> Add/2
  Product/1 -> Gain4/1
  Sin/1 -> Product/1
  We/1 -> Product/2
  Unit Delay1/1 -> Gain/1
  Unit Delay2/1 -> Subtract1/2

== system MI6FS_HE_6PhS/Phase System/Subsystem12/-wt ==
  Bias2 : Bias  Bias=-2*pi*2*50*Ts  SaturateOnIntegerOverflow=off
  Scope22 : Scope
  Unit Delay : UnitDelay  SampleTime=-1  HasFrameUpgradeWarning=on
  -wt : Outport
  wires:
  Unit Delay/1 -> Bias2/1
  Bias2/1 -> -wt/1, Scope22/1, Unit Delay/1

== system MI6FS_HE_6PhS/Phase System/Subsystem13/-wt ==
  Bias2 : Bias  Bias=-2*pi*2*50*Ts  SaturateOnIntegerOverflow=off
  Scope22 : Scope
  Unit Delay : UnitDelay  SampleTime=-1  HasFrameUpgradeWarning=on
  -wt : Outport
  wires:
  Bias2/1 -> Unit Delay/1, Scope22/1, -wt/1
  Unit Delay/1 -> Bias2/1

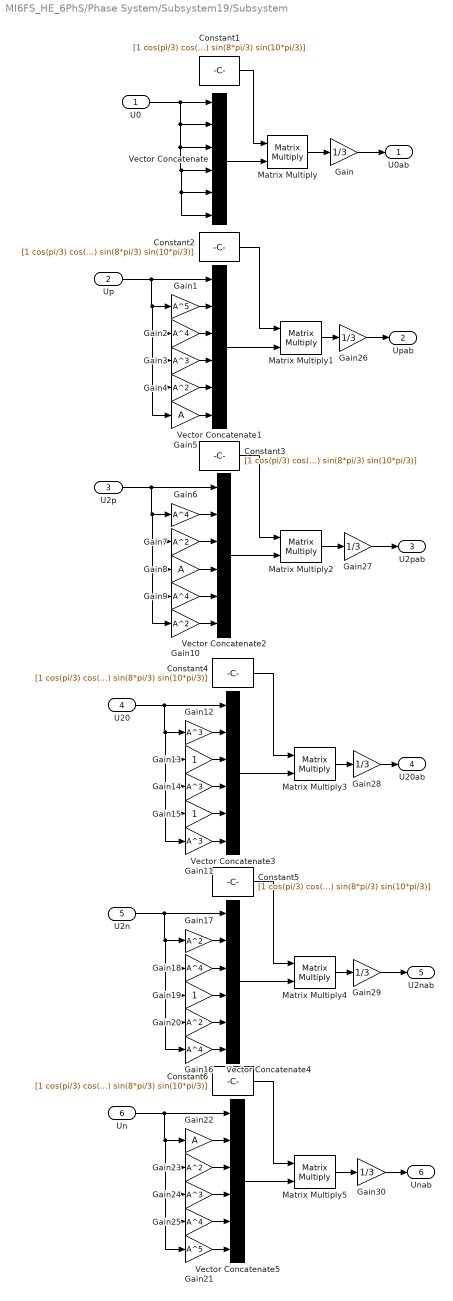
== system MI6FS_HE_6PhS/Phase System/Subsystem19/Subsystem ==
  U0 : Inport
  Up : Inport  Port=2
  U2p : Inport  Port=3
  U20 : Inport  Port=4
  U2n : Inport  Port=5
  Un : Inport  Port=6
  Constant{1..6} (6 alike) : Constant  Value=[1 cos(pi/3) cos(2*pi/3) cos(3*pi/3) cos(4*pi/3) cos(5*pi/3); 0 sin(pi/3) sin(2*pi/3) sin(3*pi/3) sin(4*pi/3) sin(5*pi/3); 1 cos(2*pi/3) cos(4*pi/3) cos(6*pi/3) cos(8*pi/3) cos(10*pi/3);1 sin(2*pi/3) sin(4*pi/3) sin(6*pi/3) sin(8*pi/3) sin(10*pi/3)]
  Gain{,26..30} (6 alike) : Gain  Gain=1/3
  Gain1 : Gain  Gain=A^5
  Gain{4,7,10,17,20,23} (6 alike) : Gain  Gain=A^2
  Gain{3,11..12,14,24} (5 alike) : Gain  Gain=A^3
  Gain13 : Gain
  Gain15 : Gain
  Gain{2,6,9,16,18,25} (6 alike) : Gain  Gain=A^4
  Gain19 : Gain
  Gain21 : Gain  Gain=A^5
  Gain22 : Gain  Gain=A
  Gain5 : Gain  Gain=A
  Gain8 : Gain  Gain=A
  Matrix Multiply{,1..5} (6 alike) : Product  Multiplication=Matrix(*)
  Vector Concatenate{,1..5} (6 alike) : Concatenate  NumInputs=6
  U0ab : Outport
  Upab : Outport  Port=2
  U2pab : Outport  Port=3
  U20ab : Outport  Port=4
  U2nab : Outport  Port=5
  Unab : Outport  Port=6
  wires:
  U0/1 -> Vector Concatenate/1, Vector Concatenate/2, Vector Concatenate/3, Vector Concatenate/4, Vector Concatenate/6, Vector Concatenate/5
  Vector Concatenate/1 -> Matrix Multiply/2
  Constant1/1 -> Matrix Multiply/1
  Matrix Multiply/1 -> Gain/1
  Up/1 -> Gain5/1, Gain4/1, Gain3/1, Gain2/1, Gain1/1, Vector Concatenate1/1
  Gain1/1 -> Vector Concatenate1/2
  Gain2/1 -> Vector Concatenate1/3
  Gain3/1 -> Vector Concatenate1/4
  Gain4/1 -> Vector Concatenate1/5
  Gain5/1 -> Vector Concatenate1/6
  Vector Concatenate1/1 -> Matrix Multiply1/2
  Constant2/1 -> Matrix Multiply1/1
  Gain8/1 -> Vector Concatenate2/4
  Gain6/1 -> Vector Concatenate2/2
  Gain9/1 -> Vector Concatenate2/5
  Gain10/1 -> Vector Concatenate2/6
  Constant3/1 -> Matrix Multiply2/1
  U2p/1 -> Vector Concatenate2/1, Gain10/1, Gain9/1, Gain8/1, Gain7/1, Gain6/1
  Gain7/1 -> Vector Concatenate2/3
  Vector Concatenate2/1 -> Matrix Multiply2/2
  Gain13/1 -> Vector Concatenate3/3
  Vector Concatenate3/1 -> Matrix Multiply3/2
  U20/1 -> Vector Concatenate3/1, Gain11/1, Gain15/1, Gain14/1, Gain13/1, Gain12/1
  Gain15/1 -> Vector Concatenate3/5
  Gain12/1 -> Vector Concatenate3/2
  Constant4/1 -> Matrix Multiply3/1
  Gain14/1 -> Vector Concatenate3/4
  Gain11/1 -> Vector Concatenate3/6
  Gain17/1 -> Vector Concatenate4/2
  Gain16/1 -> Vector Concatenate4/6
  Constant5/1 -> Matrix Multiply4/1
  Gain20/1 -> Vector Concatenate4/5
  U2n/1 -> Vector Concatenate4/1, Gain16/1, Gain20/1, Gain19/1, Gain18/1, Gain17/1
  Vector Concatenate4/1 -> Matrix Multiply4/2
  Gain19/1 -> Vector Concatenate4/4
  Gain18/1 -> Vector Concatenate4/3
  Gain23/1 -> Vector Concatenate5/3
  Vector Concatenate5/1 -> Matrix Multiply5/2
  Gain24/1 -> Vector Concatenate5/4
  Gain21/1 -> Vector Concatenate5/6
  Un/1 -> Vector Concatenate5/1, Gain21/1, Gain25/1, Gain24/1, Gain23/1, Gain22/1
  Constant6/1 -> Matrix Multiply5/1
  Gain25/1 -> Vector Concatenate5/5
  Gain22/1 -> Vector Concatenate5/2
  Gain/1 -> U0ab/1
  Gain26/1 -> Upab/1
  Matrix Multiply1/1 -> Gain26/1
  Matrix Multiply2/1 -> Gain27/1
  Gain27/1 -> U2pab/1
  Gain28/1 -> U20ab/1
  Matrix Multiply3/1 -> Gain28/1
  Matrix Multiply4/1 -> Gain29/1
  Gain29/1 -> U2nab/1
  Matrix Multiply5/1 -> Gain30/1
  Gain30/1 -> Unab/1

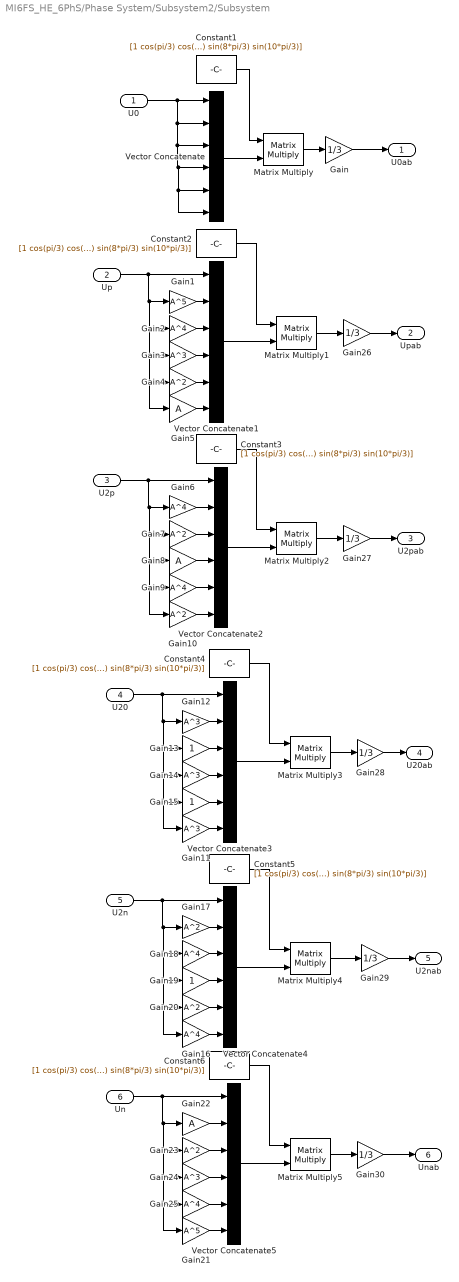
== system MI6FS_HE_6PhS/Phase System/Subsystem2/Subsystem ==
  U0 : Inport
  Up : Inport  Port=2
  U2p : Inport  Port=3
  U20 : Inport  Port=4
  U2n : Inport  Port=5
  Un : Inport  Port=6
  Constant{1..6} (6 alike) : Constant  Value=[1 cos(pi/3) cos(2*pi/3) cos(3*pi/3) cos(4*pi/3) cos(5*pi/3); 0 sin(pi/3) sin(2*pi/3) sin(3*pi/3) sin(4*pi/3) sin(5*pi/3); 1 cos(2*pi/3) cos(4*pi/3) cos(6*pi/3) cos(8*pi/3) cos(10*pi/3);1 sin(2*pi/3) sin(4*pi/3) sin(6*pi/3) sin(8*pi/3) sin(10*pi/3)]
  Gain{,26..30} (6 alike) : Gain  Gain=1/3
  Gain1 : Gain  Gain=A^5
  Gain{4,7,10,17,20,23} (6 alike) : Gain  Gain=A^2
  Gain{3,11..12,14,24} (5 alike) : Gain  Gain=A^3
  Gain13 : Gain
  Gain15 : Gain
  Gain{2,6,9,16,18,25} (6 alike) : Gain  Gain=A^4
  Gain19 : Gain
  Gain21 : Gain  Gain=A^5
  Gain22 : Gain  Gain=A
  Gain5 : Gain  Gain=A
  Gain8 : Gain  Gain=A
  Matrix Multiply{,1..5} (6 alike) : Product  Multiplication=Matrix(*)
  Vector Concatenate{,1..5} (6 alike) : Concatenate  NumInputs=6
  U0ab : Outport
  Upab : Outport  Port=2
  U2pab : Outport  Port=3
  U20ab : Outport  Port=4
  U2nab : Outport  Port=5
  Unab : Outport  Port=6
  wires:
  U0/1 -> Vector Concatenate/1, Vector Concatenate/2, Vector Concatenate/3, Vector Concatenate/4, Vector Concatenate/6, Vector Concatenate/5
  Vector Concatenate/1 -> Matrix Multiply/2
  Constant1/1 -> Matrix Multiply/1
  Matrix Multiply/1 -> Gain/1
  Up/1 -> Gain5/1, Gain4/1, Gain3/1, Gain2/1, Gain1/1, Vector Concatenate1/1
  Gain1/1 -> Vector Concatenate1/2
  Gain2/1 -> Vector Concatenate1/3
  Gain3/1 -> Vector Concatenate1/4
  Gain4/1 -> Vector Concatenate1/5
  Gain5/1 -> Vector Concatenate1/6
  Vector Concatenate1/1 -> Matrix Multiply1/2
  Constant2/1 -> Matrix Multiply1/1
  Matrix Multiply1/1 -> Gain26/1
  Gain8/1 -> Vector Concatenate2/4
  Gain6/1 -> Vector Concatenate2/2
  Gain9/1 -> Vector Concatenate2/5
  Gain10/1 -> Vector Concatenate2/6
  Constant3/1 -> Matrix Multiply2/1
  U2p/1 -> Vector Concatenate2/1, Gain10/1, Gain9/1, Gain8/1, Gain7/1, Gain6/1
  Gain7/1 -> Vector Concatenate2/3
  Matrix Multiply2/1 -> Gain27/1
  Vector Concatenate2/1 -> Matrix Multiply2/2
  Matrix Multiply3/1 -> Gain28/1
  Gain13/1 -> Vector Concatenate3/3
  Vector Concatenate3/1 -> Matrix Multiply3/2
  U20/1 -> Vector Concatenate3/1, Gain11/1, Gain15/1, Gain14/1, Gain13/1, Gain12/1
  Gain15/1 -> Vector Concatenate3/5
  Gain12/1 -> Vector Concatenate3/2
  Constant4/1 -> Matrix Multiply3/1
  Gain14/1 -> Vector Concatenate3/4
  Gain11/1 -> Vector Concatenate3/6
  Gain17/1 -> Vector Concatenate4/2
  Gain16/1 -> Vector Concatenate4/6
  Constant5/1 -> Matrix Multiply4/1
  Gain20/1 -> Vector Concatenate4/5
  U2n/1 -> Vector Concatenate4/1, Gain16/1, Gain20/1, Gain19/1, Gain18/1, Gain17/1
  Vector Concatenate4/1 -> Matrix Multiply4/2
  Gain19/1 -> Vector Concatenate4/4
  Matrix Multiply4/1 -> Gain29/1
  Gain18/1 -> Vector Concatenate4/3
  Gain23/1 -> Vector Concatenate5/3
  Vector Concatenate5/1 -> Matrix Multiply5/2
  Gain24/1 -> Vector Concatenate5/4
  Matrix Multiply5/1 -> Gain30/1
  Gain21/1 -> Vector Concatenate5/6
  Un/1 -> Vector Concatenate5/1, Gain21/1, Gain25/1, Gain24/1, Gain23/1, Gain22/1
  Constant6/1 -> Matrix Multiply5/1
  Gain25/1 -> Vector Concatenate5/5
  Gain22/1 -> Vector Concatenate5/2
  Gain/1 -> U0ab/1
  Gain26/1 -> Upab/1
  Gain27/1 -> U2pab/1
  Gain28/1 -> U20ab/1
  Gain29/1 -> U2nab/1
  Gain30/1 -> Unab/1

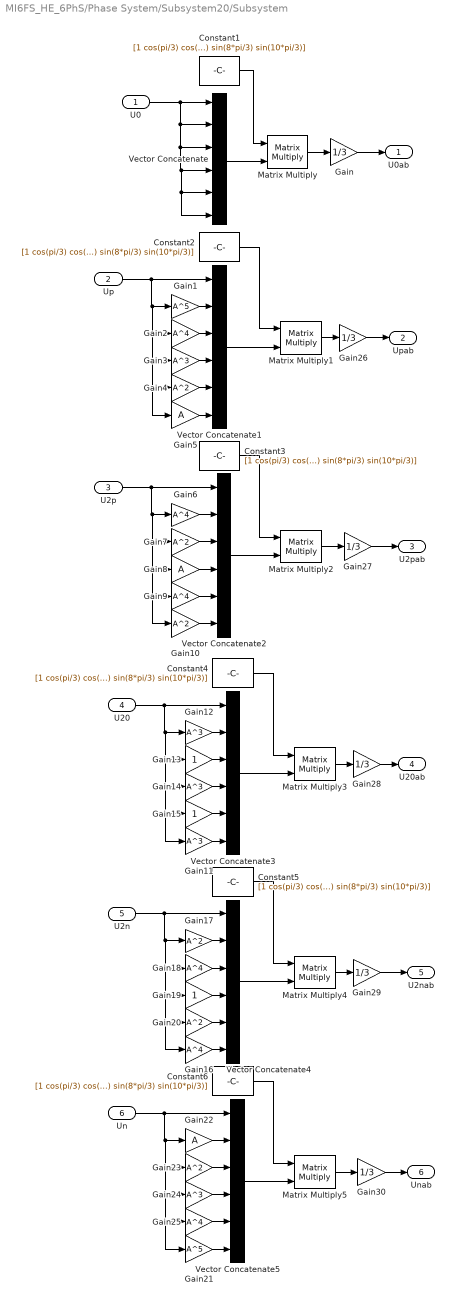
== system MI6FS_HE_6PhS/Phase System/Subsystem20/Subsystem ==
  U0 : Inport
  Up : Inport  Port=2
  U2p : Inport  Port=3
  U20 : Inport  Port=4
  U2n : Inport  Port=5
  Un : Inport  Port=6
  Constant{1..6} (6 alike) : Constant  Value=[1 cos(pi/3) cos(2*pi/3) cos(3*pi/3) cos(4*pi/3) cos(5*pi/3); 0 sin(pi/3) sin(2*pi/3) sin(3*pi/3) sin(4*pi/3) sin(5*pi/3); 1 cos(2*pi/3) cos(4*pi/3) cos(6*pi/3) cos(8*pi/3) cos(10*pi/3);1 sin(2*pi/3) sin(4*pi/3) sin(6*pi/3) sin(8*pi/3) sin(10*pi/3)]
  Gain{,26..30} (6 alike) : Gain  Gain=1/3
  Gain1 : Gain  Gain=A^5
  Gain{4,7,10,17,20,23} (6 alike) : Gain  Gain=A^2
  Gain{3,11..12,14,24} (5 alike) : Gain  Gain=A^3
  Gain13 : Gain
  Gain15 : Gain
  Gain{2,6,9,16,18,25} (6 alike) : Gain  Gain=A^4
  Gain19 : Gain
  Gain21 : Gain  Gain=A^5
  Gain22 : Gain  Gain=A
  Gain5 : Gain  Gain=A
  Gain8 : Gain  Gain=A
  Matrix Multiply{,1..5} (6 alike) : Product  Multiplication=Matrix(*)
  Vector Concatenate{,1..5} (6 alike) : Concatenate  NumInputs=6
  U0ab : Outport
  Upab : Outport  Port=2
  U2pab : Outport  Port=3
  U20ab : Outport  Port=4
  U2nab : Outport  Port=5
  Unab : Outport  Port=6
  wires:
  Gain30/1 -> Unab/1
  Matrix Multiply5/1 -> Gain30/1
  Gain29/1 -> U2nab/1
  Matrix Multiply4/1 -> Gain29/1
  Matrix Multiply3/1 -> Gain28/1
  Gain28/1 -> U20ab/1
  Gain27/1 -> U2pab/1
  Matrix Multiply2/1 -> Gain27/1
  Matrix Multiply1/1 -> Gain26/1
  Gain26/1 -> Upab/1
  Gain/1 -> U0ab/1
  Gain22/1 -> Vector Concatenate5/2
  Gain25/1 -> Vector Concatenate5/5
  Constant6/1 -> Matrix Multiply5/1
  Un/1 -> Gain22/1, Gain23/1, Gain24/1, Gain25/1, Gain21/1, Vector Concatenate5/1
  Gain21/1 -> Vector Concatenate5/6
  Gain24/1 -> Vector Concatenate5/4
  Vector Concatenate5/1 -> Matrix Multiply5/2
  Gain23/1 -> Vector Concatenate5/3
  Gain18/1 -> Vector Concatenate4/3
  Gain19/1 -> Vector Concatenate4/4
  Vector Concatenate4/1 -> Matrix Multiply4/2
  U2n/1 -> Gain17/1, Gain18/1, Gain19/1, Gain20/1, Gain16/1, Vector Concatenate4/1
  Gain20/1 -> Vector Concatenate4/5
  Constant5/1 -> Matrix Multiply4/1
  Gain16/1 -> Vector Concatenate4/6
  Gain17/1 -> Vector Concatenate4/2
  Gain11/1 -> Vector Concatenate3/6
  Gain14/1 -> Vector Concatenate3/4
  Constant4/1 -> Matrix Multiply3/1
  Gain12/1 -> Vector Concatenate3/2
  Gain15/1 -> Vector Concatenate3/5
  U20/1 -> Gain12/1, Gain13/1, Gain14/1, Gain15/1, Gain11/1, Vector Concatenate3/1
  Vector Concatenate3/1 -> Matrix Multiply3/2
  Gain13/1 -> Vector Concatenate3/3
  Vector Concatenate2/1 -> Matrix Multiply2/2
  Gain7/1 -> Vector Concatenate2/3
  U2p/1 -> Gain6/1, Gain7/1, Gain8/1, Gain9/1, Gain10/1, Vector Concatenate2/1
  Constant3/1 -> Matrix Multiply2/1
  Gain10/1 -> Vector Concatenate2/6
  Gain9/1 -> Vector Concatenate2/5
  Gain6/1 -> Vector Concatenate2/2
  Gain8/1 -> Vector Concatenate2/4
  Constant2/1 -> Matrix Multiply1/1
  Vector Concatenate1/1 -> Matrix Multiply1/2
  Gain5/1 -> Vector Concatenate1/6
  Gain4/1 -> Vector Concatenate1/5
  Gain3/1 -> Vector Concatenate1/4
  Gain2/1 -> Vector Concatenate1/3
  Gain1/1 -> Vector Concatenate1/2
  Up/1 -> Vector Concatenate1/1, Gain1/1, Gain2/1, Gain3/1, Gain4/1, Gain5/1
  Matrix Multiply/1 -> Gain/1
  Constant1/1 -> Matrix Multiply/1
  Vector Concatenate/1 -> Matrix Multiply/2
  U0/1 -> Vector Concatenate/5, Vector Concatenate/6, Vector Concatenate/4, Vector Concatenate/3, Vector Concatenate/2, Vector Concatenate/1
